simulink model "integrator"  (R2020a)
settings: Solver=VariableStepAuto  StartTime=0.0  StopTime=10  RelTol=1e-3
settings Model: Creator=RaviM  LastModifiedBy=RaviM

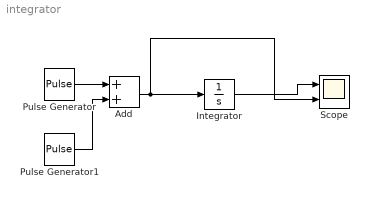
== system integrator ==
  Add : Sum
  Integrator : Integrator
  Pulse Generator : DiscretePulseGenerator  PulseType=Time based  Amplitude=10  Period=10  PulseWidth=50
  Pulse Generator1 : DiscretePulseGenerator  PulseType=Time based  Amplitude=-10  Period=10  PulseWidth=50  PhaseDelay=5
  Scope : Scope  NumInputPorts=2
  wires:
  Pulse Generator/1 -> Add/1
  Pulse Generator1/1 -> Add/2
  Add/1 -> Integrator/1, Scope/2
  Integrator/1 -> Scope/1
